simulink model "IDctrl"  (R2018b)
settings: Solver=FixedStepAuto  StartTime=0.0  StopTime=tfin  FixedStep=timeStep  MaxStep=1e-4  RelTol=1e-3
InitFcn:
  | initSim=true;
  | initIDctrl
StopFcn:
  | initSim=false;
  | initIDctrl
values from neighbouring files (symbols this model uses):
  kd = wn*damp*2    (= 28.5)    [es_1_circle.m]    (also in es_1_line.m = 57; initIDctrl.m = 32)
  kp = wn^2    (= 225)    [es_1_circle.m]    (also in es_1_line.m = 900; initIDctrl.m = 400)
libraries: roblocks x4
settings Model: Creator=Brus  LastModifiedBy=Brus

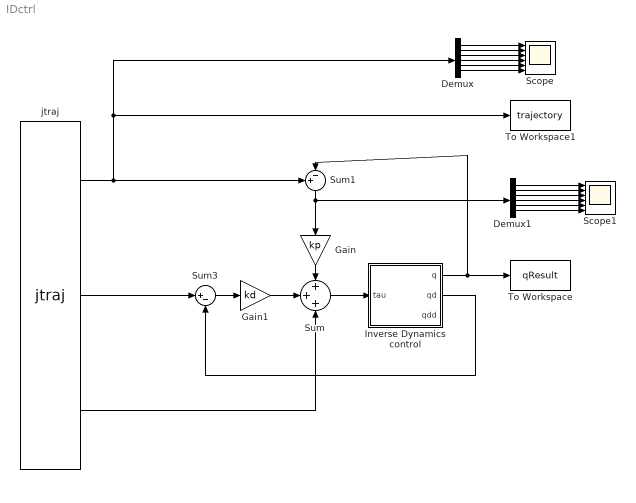
== system IDctrl ==
  Demux : Demux  Outputs=6
  Demux1 : Demux  Outputs=6
  Gain : Gain  Gain=kp
  Gain1 : Gain  Gain=kd
  Inverse Dynamics control : Subsystem
  Scope : Scope  NumInputPorts=6
  Scope1 : Scope  NumInputPorts=6
  Sum : Sum  Inputs=+++
  Sum1 : Sum  Inputs=+-|
  Sum3 : Sum  Inputs=|+-
  To Workspace : ToWorkspace  VariableName=qResult  SaveFormat=Timeseries  SampleTime=-1
  To Workspace1 : ToWorkspace  VariableName=trajectory  SaveFormat=Timeseries  SampleTime=-1
  jtraj : roblocks/Toolbox/jtraj  q0=q0  qf=qf  tmax=tfin  ts=trajStep
  wires:
  Gain/1 -> Sum/1
  Gain1/1 -> Sum/2
  Sum3/1 -> Gain1/1
  Sum1/1 -> Gain/1, Demux1/1
  Sum/1 -> Inverse Dynamics control/1(tau)
  Inverse Dynamics control/2(qd) -> Sum3/2
  jtraj/2 -> Sum3/1
  jtraj/3 -> Sum/3
  Demux/5 -> Scope/5
  Demux/1 -> Scope/1
  Demux/6 -> Scope/6
  Demux/2 -> Scope/2
  Demux/3 -> Scope/3
  jtraj/1 -> Demux/1, To Workspace1/1, Sum1/1
  Demux/4 -> Scope/4
  Demux1/5 -> Scope1/5
  Demux1/1 -> Scope1/1
  Demux1/6 -> Scope1/6
  Demux1/2 -> Scope1/2
  Demux1/3 -> Scope1/3
  Inverse Dynamics control/1(q) -> To Workspace/1, Sum1/2
  Demux1/4 -> Scope1/4

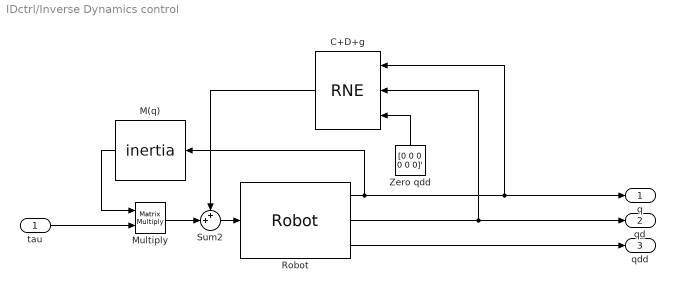
== system IDctrl/Inverse Dynamics control ==
  tau : Inport
  C+D+g : roblocks/Arm/RNE  robot=p560_canc  grav=[0 0 9.81]
  M(q) : roblocks/Arm/inertia  robot=p560_canc
  Multiply : Product  Multiplication=Matrix(*)
  Robot : roblocks/Arm/Robot  robot=p560  q0=q0
  Sum2 : Sum  Inputs=++|
  Zero qdd : Constant  Value=[0 0 0 0 0 0]'
  q : Outport
  qd : Outport  Port=2
  qdd : Outport  Port=3
  wires:
  Multiply/1 -> Sum2/2
  Sum2/1 -> Robot/1
  Zero qdd/1 -> C+D+g/3
  Robot/1 -> q/1, C+D+g/1, M(q)/1
  M(q)/1 -> Multiply/1
  C+D+g/1 -> Sum2/1
  Robot/2 -> qd/1, C+D+g/2
  tau/1 -> Multiply/2
  Robot/3 -> qdd/1
